simulink model "ccp_slave_demo"  (Simulink 7.3)
settings: Solver=ode3  SolverMode=SingleTasking  StartTime=0.0  StopTime=10.0  RelTol=1e-3
PreLoadFcn:
  | waijung.modelPreload; % Required for working with Waijung Blockset. Do not remove.
undefined symbols (not defined in the file): LQFP48, STM32F072CB
libraries: simulink x216, waijung_soft_i2c_lib x28, waijung_addon_module x12, stm32f0_flash_lib x10, stm32f0_can_lib x3, stm32f0_reset_lib x1, waijung_crc_lib x1, stm32f0_device_config_lib x1
(part 6 of 6)

== system ccp_slave_demo/CCP Handler/Command Processing/UPLOAD/UPLOAD/UPLOAD/MEM_EEPROM/Subsystem ==
  In1 : Inport
  Enable : EnablePort
  Compare To Zero : simulink/Logic and Bit Operations/Compare To Zero  SystemSampleTime=-1  relop===  LogicOutDataTypeMode=uint8  ZeroCross=off
  Constant : Constant  Value=0  OutDataTypeMode=uint8  OutDataType=fixdt(1, 16)  OutScaling=2^0  OutDataTypeStr=uint8
  Constant1 : Constant  Value=hex2dec('A0')  OutDataTypeMode=uint8  OutDataType=fixdt(1, 16)  OutScaling=2^0  OutDataTypeStr=uint8
  Data Type Conversion : DataTypeConversion  OutDataType=fixdt(1, 16)  OutScaling=2^0
  Mux : Mux  Inputs=5
  Soft I2C Master Read/Write : waijung_soft_i2c_lib/Soft I2C Master Read//Write  conf=ReadWrite  targetname=stm32f0  module=1  transfer=Blocking  clk=100  timeout=25  sdapins={'A4','A6'}  sclpins='A5'  writecount=1  readcount=1  waittime=0  forcestop=off  portpinstr=0  sampletime=inf  blockid=CCPHandlerCommandProcessingUPLOADUPLOADUPLOADMEM_EEPROMSubsystemSoftI2CMasterReadWrite  inputporttype=[3 3]  inputportwidth=[]  inputportlabel={'SlvAddr' 'Wr0 (uint8)'}  outputporttype=[3 3 ]  outputportwidth=[1 1]  outputportlabel={'Status' 'Rd0 (uint8)'}  compat=0  optionstring="[\"1\",\"1\",\"1\",\"0\",\"off\",\"1\"]"
  Valid : Outport
  Out : Outport  Port=2  InitialOutput=[0 0 0 0 0]
  wires:
  Constant1/1 -> Soft I2C Master Read/Write/1
  Data Type Conversion/1 -> Soft I2C Master Read/Write/2
  Soft I2C Master Read/Write/1 -> Compare To Zero/1
  In1/1 -> Data Type Conversion/1
  Compare To Zero/1 -> Valid/1
  Soft I2C Master Read/Write/2 -> Mux/1
  Mux/1 -> Out/1
  Constant/1 -> Mux/3, Mux/2, Mux/4, Mux/5

== system ccp_slave_demo/CCP Handler/Command Processing/UPLOAD/UPLOAD/UPLOAD/MEM_EEPROM/Subsystem1 ==
  In1 : Inport
  Enable : EnablePort
  Compare To Zero : simulink/Logic and Bit Operations/Compare To Zero  SystemSampleTime=-1  relop===  LogicOutDataTypeMode=uint8  ZeroCross=off
  Constant : Constant  Value=0  OutDataTypeMode=uint8  OutDataType=fixdt(1, 16)  OutScaling=2^0  OutDataTypeStr=uint8
  Constant1 : Constant  Value=hex2dec('A0')  OutDataTypeMode=uint8  OutDataType=fixdt(1, 16)  OutScaling=2^0  OutDataTypeStr=uint8
  Data Type Conversion : DataTypeConversion  OutDataType=fixdt(1, 16)  OutScaling=2^0
  Mux : Mux  Inputs=5
  Soft I2C Master Read/Write : waijung_soft_i2c_lib/Soft I2C Master Read//Write  conf=ReadWrite  targetname=stm32f0  module=1  transfer=Blocking  clk=100  timeout=25  sdapins={'A4','A6'}  sclpins='A5'  writecount=1  readcount=2  waittime=0  forcestop=off  portpinstr=0  sampletime=inf  blockid=CCPHandlerCommandProcessingUPLOADUPLOADUPLOADMEM_EEPROMSubsystem1SoftI2CMasterReadWrite  inputporttype=[3 3]  inputportwidth=[]  inputportlabel={'SlvAddr' 'Wr0 (uint8)'}  outputporttype="[3 3 3  ]"  outputportwidth=[1 1 1]  outputportlabel={'Status' 'Rd0 (uint8)' 'Rd1 (uint8)'}  compat=0  optionstring="[\"1\",\"1\",\"2\",\"0\",\"off\",\"1\"]"
  Valid : Outport
  Out : Outport  Port=2  InitialOutput=[0 0 0 0 0]
  wires:
  Mux/1 -> Out/1
  Soft I2C Master Read/Write/2 -> Mux/1
  Compare To Zero/1 -> Valid/1
  In1/1 -> Data Type Conversion/1
  Soft I2C Master Read/Write/1 -> Compare To Zero/1
  Data Type Conversion/1 -> Soft I2C Master Read/Write/2
  Constant1/1 -> Soft I2C Master Read/Write/1
  Soft I2C Master Read/Write/3 -> Mux/2
  Constant/1 -> Mux/4, Mux/3, Mux/5

== system ccp_slave_demo/CCP Handler/Command Processing/UPLOAD/UPLOAD/UPLOAD/MEM_EEPROM/Subsystem2 ==
  In1 : Inport
  Enable : EnablePort
  Compare To Zero : simulink/Logic and Bit Operations/Compare To Zero  SystemSampleTime=-1  relop===  LogicOutDataTypeMode=uint8  ZeroCross=off
  Constant : Constant  Value=0  OutDataTypeMode=uint8  OutDataType=fixdt(1, 16)  OutScaling=2^0  OutDataTypeStr=uint8
  Constant1 : Constant  Value=hex2dec('A0')  OutDataTypeMode=uint8  OutDataType=fixdt(1, 16)  OutScaling=2^0  OutDataTypeStr=uint8
  Data Type Conversion : DataTypeConversion  OutDataType=fixdt(1, 16)  OutScaling=2^0
  Mux : Mux  Inputs=5
  Soft I2C Master Read/Write : waijung_soft_i2c_lib/Soft I2C Master Read//Write  conf=ReadWrite  targetname=stm32f0  module=1  transfer=Blocking  clk=100  timeout=25  sdapins={'A4','A6'}  sclpins='A5'  writecount=1  readcount=3  waittime=0  forcestop=off  portpinstr=0  sampletime=inf  blockid=CCPHandlerCommandProcessingUPLOADUPLOADUPLOADMEM_EEPROMSubsystem2SoftI2CMasterReadWrite  inputporttype=[3 3]  inputportwidth=[]  inputportlabel={'SlvAddr' 'Wr0 (uint8)'}  outputporttype="[3 3 3 3   ]"  outputportwidth=[1 1 1 1]  outputportlabel={'Status' 'Rd0 (uint8)' 'Rd1 (uint8)' 'Rd2 (uint8)'}  compat=0  optionstring="[\"1\",\"1\",\"3\",\"0\",\"off\",\"1\"]"
  Valid : Outport
  Out : Outport  Port=2  InitialOutput=[0 0 0 0 0]
  wires:
  Soft I2C Master Read/Write/3 -> Mux/2
  Constant1/1 -> Soft I2C Master Read/Write/1
  Data Type Conversion/1 -> Soft I2C Master Read/Write/2
  Soft I2C Master Read/Write/1 -> Compare To Zero/1
  In1/1 -> Data Type Conversion/1
  Compare To Zero/1 -> Valid/1
  Soft I2C Master Read/Write/2 -> Mux/1
  Mux/1 -> Out/1
  Soft I2C Master Read/Write/4 -> Mux/3
  Constant/1 -> Mux/4, Mux/5

== system ccp_slave_demo/CCP Handler/Command Processing/UPLOAD/UPLOAD/UPLOAD/MEM_EEPROM/Subsystem3 ==
  In1 : Inport
  Enable : EnablePort
  Compare To Zero : simulink/Logic and Bit Operations/Compare To Zero  SystemSampleTime=-1  relop===  LogicOutDataTypeMode=uint8  ZeroCross=off
  Constant : Constant  Value=0  OutDataTypeMode=uint8  OutDataType=fixdt(1, 16)  OutScaling=2^0  OutDataTypeStr=uint8
  Constant1 : Constant  Value=hex2dec('A0')  OutDataTypeMode=uint8  OutDataType=fixdt(1, 16)  OutScaling=2^0  OutDataTypeStr=uint8
  Data Type Conversion : DataTypeConversion  OutDataType=fixdt(1, 16)  OutScaling=2^0
  Mux : Mux  Inputs=5
  Soft I2C Master Read/Write : waijung_soft_i2c_lib/Soft I2C Master Read//Write  conf=ReadWrite  targetname=stm32f0  module=1  transfer=Blocking  clk=100  timeout=25  sdapins={'A4','A6'}  sclpins='A5'  writecount=1  readcount=4  waittime=0  forcestop=off  portpinstr=0  sampletime=inf  blockid=CCPHandlerCommandProcessingUPLOADUPLOADUPLOADMEM_EEPROMSubsystem3SoftI2CMasterReadWrite  inputporttype=[3 3]  inputportwidth=[]  inputportlabel={'SlvAddr' 'Wr0 (uint8)'}  outputporttype="[3 3 3 3 3    ]"  outputportwidth=[1 1 1 1 1]  outputportlabel={'Status' 'Rd0 (uint8)' 'Rd1 (uint8)' 'Rd2 (uint8)' 'Rd3 (uint8)'}  compat=0  optionstring="[\"1\",\"1\",\"4\",\"0\",\"off\",\"1\"]"
  Valid : Outport
  Out : Outport  Port=2  InitialOutput=[0 0 0 0 0]
  wires:
  Soft I2C Master Read/Write/4 -> Mux/3
  Mux/1 -> Out/1
  Soft I2C Master Read/Write/2 -> Mux/1
  Compare To Zero/1 -> Valid/1
  In1/1 -> Data Type Conversion/1
  Soft I2C Master Read/Write/1 -> Compare To Zero/1
  Data Type Conversion/1 -> Soft I2C Master Read/Write/2
  Constant1/1 -> Soft I2C Master Read/Write/1
  Soft I2C Master Read/Write/3 -> Mux/2
  Constant/1 -> Mux/5
  Soft I2C Master Read/Write/5 -> Mux/4

== system ccp_slave_demo/CCP Handler/Command Processing/UPLOAD/UPLOAD/UPLOAD/MEM_EEPROM/Subsystem4 ==
  In1 : Inport
  Enable : EnablePort
  Compare To Zero : simulink/Logic and Bit Operations/Compare To Zero  SystemSampleTime=-1  relop===  LogicOutDataTypeMode=uint8  ZeroCross=off
  Constant1 : Constant  Value=hex2dec('A0')  OutDataTypeMode=uint8  OutDataType=fixdt(1, 16)  OutScaling=2^0  OutDataTypeStr=uint8
  Data Type Conversion : DataTypeConversion  OutDataType=fixdt(1, 16)  OutScaling=2^0
  Mux : Mux  Inputs=5
  Soft I2C Master Read/Write : waijung_soft_i2c_lib/Soft I2C Master Read//Write  conf=ReadWrite  targetname=stm32f0  module=1  transfer=Blocking  clk=100  timeout=25  sdapins={'A4','A6'}  sclpins='A5'  writecount=1  readcount=5  waittime=0  forcestop=off  portpinstr=0  sampletime=inf  blockid=CCPHandlerCommandProcessingUPLOADUPLOADUPLOADMEM_EEPROMSubsystem4SoftI2CMasterReadWrite  inputporttype=[3 3]  inputportwidth=[]  inputportlabel={'SlvAddr' 'Wr0 (uint8)'}  outputporttype="[3 3 3 3 3 3     ]"  outputportwidth=[1 1 1 1 1 1]  outputportlabel={'Status' 'Rd0 (uint8)' 'Rd1 (uint8)' 'Rd2 (uint8)' 'Rd3 (uint8)' 'Rd4 (uint8)'}  compat=0  optionstring="[\"1\",\"1\",\"5\",\"0\",\"off\",\"1\"]"
  Valid : Outport
  Out : Outport  Port=2  InitialOutput=[0 0 0 0 0]
  wires:
  Soft I2C Master Read/Write/5 -> Mux/4
  Soft I2C Master Read/Write/6 -> Mux/5
  Soft I2C Master Read/Write/3 -> Mux/2
  Constant1/1 -> Soft I2C Master Read/Write/1
  Data Type Conversion/1 -> Soft I2C Master Read/Write/2
  Soft I2C Master Read/Write/1 -> Compare To Zero/1
  In1/1 -> Data Type Conversion/1
  Compare To Zero/1 -> Valid/1
  Soft I2C Master Read/Write/2 -> Mux/1
  Mux/1 -> Out/1
  Soft I2C Master Read/Write/4 -> Mux/3

== system ccp_slave_demo/CCP Handler/Command Processing/UPLOAD/UPLOAD/UPLOAD/MEM_FLASH/Read Flash 2 Byte ==
  Offset : Inport  OutDataType=fixdt(1, 16)  OutScaling=2^0
  Enable : EnablePort
  Constant : Constant  Value=0  OutDataTypeMode=uint8  OutDataType=fixdt(1, 16)  OutScaling=2^0  OutDataTypeStr=uint8
  Data Type Conversion : DataTypeConversion  OutDataTypeMode=uint8  OutDataType=fixdt(1, 16)  OutScaling=2^0  OutDataTypeStr=uint8
  Data Type Conversion1 : DataTypeConversion  OutDataTypeMode=uint8  OutDataType=fixdt(1, 16)  OutScaling=2^0  OutDataTypeStr=uint8
  FLASH Read : stm32f0_flash_lib/FLASH Read  conf=Read  startaddress=0x8011000  pagesize=2k  datatype=uint16  enablestatus=off  sampletime=inf  filename='ccp_slave_demo.flash'  enablecustomportlabel=off  cinputportlabel=0  portpinstr=0  blockid=CCPHandlerCommandProcessingUPLOADUPLOADUPLOADMEM_FLASHReadFlash2ByteFLASHRead  inputporttype=[7]  inputportwidth=[]  inputportlabel={'Offset'}  outputporttype=[5]  outputportwidth=[]  outputportlabel={'Data'}  compat=0  optionstring="[\"8011000\",\"0\"]"
  Mux : Mux  Inputs=5
  Shift Arithmetic : simulink/Logic and Bit Operations/Shift Arithmetic  SystemSampleTime=-1  nBitShiftRight=8  nBinPtShiftRight=0
  Out1 : Outport  OutDataType=fixdt(1, 16)  OutScaling=2^0
  wires:
  Mux/1 -> Out1/1
  Shift Arithmetic/1 -> Data Type Conversion/1
  FLASH Read/1 -> Shift Arithmetic/1, Data Type Conversion1/1
  Offset/1 -> FLASH Read/1
  Data Type Conversion/1 -> Mux/2
  Data Type Conversion1/1 -> Mux/1
  Constant/1 -> Mux/3, Mux/4, Mux/5

== system ccp_slave_demo/CCP Handler/Command Processing/UPLOAD/UPLOAD/UPLOAD/MEM_FLASH/Read Flash 4 Byte ==
  In1 : Inport  OutDataType=fixdt(1, 16)  OutScaling=2^0
  Enable : EnablePort
  Constant : Constant  Value=0  OutDataTypeMode=uint8  OutDataType=fixdt(1, 16)  OutScaling=2^0  OutDataTypeStr=uint8
  Data Type Conversion{,1..3} (4 alike) : DataTypeConversion  OutDataTypeMode=uint8  OutDataType=fixdt(1, 16)  OutScaling=2^0  OutDataTypeStr=uint8
  FLASH Read : stm32f0_flash_lib/FLASH Read  conf=Read  startaddress=0x8011000  pagesize=2k  datatype=uint32  enablestatus=off  sampletime=inf  filename='ccp_slave_demo.flash'  enablecustomportlabel=off  cinputportlabel=0  portpinstr=0  blockid=CCPHandlerCommandProcessingUPLOADUPLOADUPLOADMEM_FLASHReadFlash4ByteFLASHRead  inputporttype=[7]  inputportwidth=[]  inputportlabel={'Offset'}  outputporttype=[7]  outputportwidth=[]  outputportlabel={'Data'}  compat=0  optionstring="[\"8011000\",\"0\"]"
  Mux : Mux  Inputs=5
  Shift Arithmetic : simulink/Logic and Bit Operations/Shift Arithmetic  SystemSampleTime=-1  nBitShiftRight=8  nBinPtShiftRight=0
  Shift Arithmetic1 : simulink/Logic and Bit Operations/Shift Arithmetic  SystemSampleTime=-1  nBitShiftRight=16  nBinPtShiftRight=0
  Shift Arithmetic2 : simulink/Logic and Bit Operations/Shift Arithmetic  SystemSampleTime=-1  nBitShiftRight=24  nBinPtShiftRight=0
  Out1 : Outport  OutDataType=fixdt(1, 16)  OutScaling=2^0
  wires:
  Mux/1 -> Out1/1
  Shift Arithmetic/1 -> Data Type Conversion/1
  FLASH Read/1 -> Shift Arithmetic/1, Data Type Conversion1/1, Shift Arithmetic1/1, Shift Arithmetic2/1
  Data Type Conversion/1 -> Mux/2
  Data Type Conversion1/1 -> Mux/1
  Shift Arithmetic1/1 -> Data Type Conversion2/1
  Data Type Conversion2/1 -> Mux/3
  Shift Arithmetic2/1 -> Data Type Conversion3/1
  Data Type Conversion3/1 -> Mux/4
  Constant/1 -> Mux/5
  In1/1 -> FLASH Read/1
